simulink model "TCMSSystem"  (R2019b)
settings: configuration reference "ConfigSet_TCMSSystem_Reference" (kept outside this file)
model workspace (MAT data in the model file):
  Prm_TCMSSystem : Simulink.Parameter (value not decoded)
  SampleTime = 0.05
symbols that are objects in the model workspace (value not decoded): Prm_TCMSSystem
undefined symbols (not defined in the file): ADDIntervention, AK1Status, AK2Status, AKContactorStatus, AllDoorsClosed, AllLeftDoorsClosed, AllRightDoorsClosed, APS1Fault, APS1Isolated, APS1OutputVoltage, APS1Status, APS2Fault, APS2Isolated, APS2OutputVoltage, APS2Status, APSKAKContactor, ASCOEnd1, ASCOEnd2, ATBMode, ATCBypassMode, ATCStatusNotOK, ATOMode, ATPLowSpeedCutoutStatus, ATPMode, AuxCompressor, BatteryCurrent, BatteryIsolationContactor, BatteryTemperature, BatteryVoltage, BCG1Fault, BCG1Isolated, BCG1IsolationFailed, BCG1OutputCurrent, BCG1Status, BCG2Fault, BCG2Isolated, BCG2OutputCurrent, BCG2Status, BCGOutputVoltage, BECU1AxleLockedWheelSet1, BECU2AxleLockedWheelSet2, BECUFaulty, BECUMajorFault, BECUMinorFault, BECUStatus, BIC1Inside, BIC1Outside, BIC2Inside, BIC2Outside, Bogie, Bogie1WSPStatus, Bogie2WSPStatus, BogieFaulty, BogieIsolationStatus, BogieSupportedMass, BrakeCylinderPressureGauge, BrakeLoopCBTripped, BrakeLoopOpenTL, BrakeTrainLineStatus, BrakingDemand ... (+215)
libraries: TimersLib x257, simulink x137, LatchesLib x42, VectorOperationsLib x15, TestBenchLib x12, MathOperationsLib x2, FiltersLib x1
(part 3 of 16)

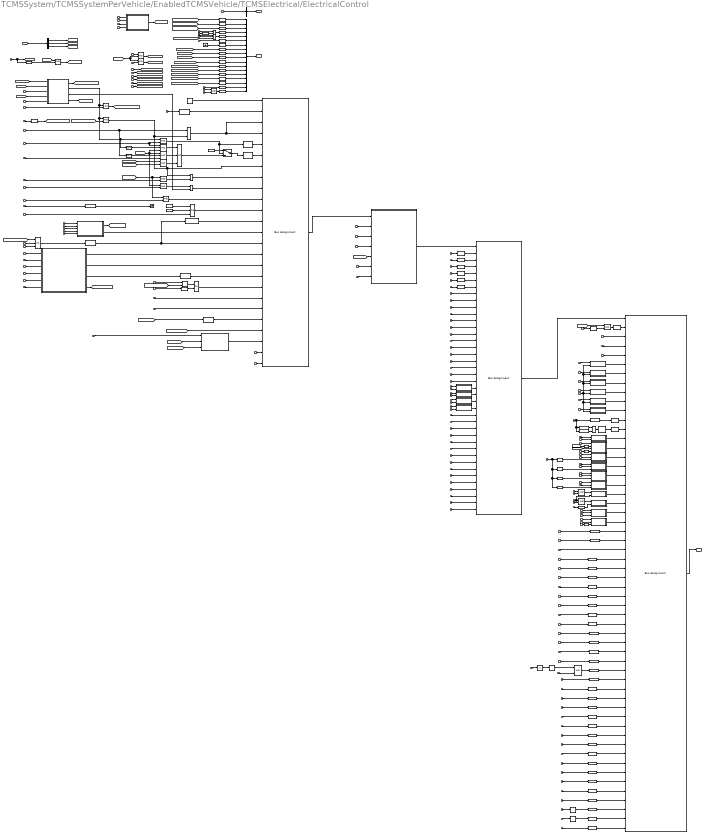
== system TCMSSystem/TCMSSystemPerVehicle/EnabledTCMSVehicle/TCMSElectrical/ElectricalControl ==
  note: Headlight High/Low:
      | Emergency Door Opened
      | Forward direction in UTO Mode
  note: Door Operations
  note: VDUInputs
  note: Fault Message Triggers
  note: Taillight White:
      | In the direction of travel
      | With Mode Selector not in OFF or Standby
  note: Taillight Red:
      | In the opposite direction of travel
      | Emergency door opened at other end
      | In Standstill at both end
  note: Floodlight:
      | Forward direction in UTO Mode
  note: Flashlight:
      | Forward direction in UTO Mode
      | While in RM mode, on the other end
  note: UTO/RM:
      | While in RM mode, on the other end
  note: Call on Light:
      | On the other end
  In Bus Element5 : Inport  PortName=WireStates  Element=TractionBrakingTrainWire.Overspeed
  In Bus Element129 : Inport  PortName=WireStates  Element=ElectricalTrainWire
  In Bus Element12 : Inport  PortName=WireStates  Element=ElectricalTrainWire.TW_EnergizeTLWRFb
  In Bus Element13 : Inport  PortName=WireStates  Element=ElectricalTrainWire.TW_RMF_RMRFb
  In Bus Element6 : Inport  PortName=WireStates  Element=ElectricalTrainWire.TW_PantoDownCmdTrip
  In Bus Element9 : Inport  PortName=WireStates  Element=ElectricalTrainWire.TW_TPOR
  In Bus Element18 : Inport  PortName=WireStates  Element=ElectricalTrainWire.TW_ATPFb
  In Bus Element25 : Inport  PortName=WireStates  Element=ElectricalTrainWire.TW_HLSwitchStatus
  In Bus Element28 : Inport  PortName=WireStates  Element=ElectricalTrainWire.TW_EmerDoorOpened
  In Bus Element26 : Inport  PortName=WireStates  Element=ElectricalTrainWire.TW_CallOnLightStatus
  In Bus Element31 : Inport  PortName=WireStates  Element=ElectricalTrainWire.TW_ZeroSpeed
  In Bus Element32 : Inport  PortName=WireStates  Element=ElectricalTrainWire.TW_UTOModeActive
  In Bus Element34 : Inport  PortName=WireStates  Element=ElectricalTrainWire.TW_DriverModeSelection
  In Bus Element128 : Inport  PortName=WireStates  Element=ElectricalTrainWire.TW_POFFPB
  In Bus Element127 : Inport  PortName=WireStates  Element=ElectricalTrainWire.TW_POFFPB
  In Bus Element130 : Inport  PortName=WireStates  Element=ElectricalTrainWire.TW_ReverseDirection
  In Bus Element132 : Inport  PortName=WireStates  Element=ElectricalTrainWire.TW_KeySwitchStatus
  In Bus Element126 : Inport  PortName=WireStates  Element=ElectricalTrainWire.TW_ShutdownFailure
  In Bus Element153 : Inport  PortName=WireStates  Element=PneumaticTrainSum.NoOfBogieIsolated
  In Bus Element125 : Inport  Port=2  PortName=CBTC
  In Bus Element33 : Inport  Port=2  PortName=CBTC  Element=DriverModeSelection
  In Bus Element45 : Inport  Port=2  PortName=CBTC  Element=ATCWakeup
  In Bus Element124 : Inport  Port=3  PortName=ElectricalSignals
  In Bus Element3 : Inport  Port=3  PortName=ElectricalSignals  Element=CabActive
  In Bus Element114 : Inport  Port=3  PortName=ElectricalSignals  Element=CabActive
  In Bus Element2 : Inport  Port=3  PortName=ElectricalSignals  Element=ZeroSpeed
  In Bus Element7 : Inport  Port=3  PortName=ElectricalSignals  Element=PowerONPBPressed
  In Bus Element8 : Inport  Port=3  PortName=ElectricalSignals  Element=PowerOFFPBPressed
  In Bus Element19 : Inport  Port=3  PortName=ElectricalSignals  Element=ForwardDirection
  In Bus Element22 : Inport  Port=3  PortName=ElectricalSignals  Element=ReverseDirection
  In Bus Element23 : Inport  Port=3  PortName=ElectricalSignals  Element=HLSwitchStatus
  In Bus Element29 : Inport  Port=3  PortName=ElectricalSignals  Element=FlasherLightStatus
  In Bus Element30 : Inport  Port=3  PortName=ElectricalSignals  Element=CallOnLightStatus
  In Bus Element16 : Inport  Port=3  PortName=ElectricalSignals  Element=PADRStatus
  In Bus Element87 : Inport  Port=3  PortName=ElectricalSignals  Element=PADRStatus
  In Bus Element17 : Inport  Port=3  PortName=ElectricalSignals  Element=ParkBrakeApplication
  In Bus Element48 : Inport  Port=3  PortName=ElectricalSignals  Element=BatteryVoltage
  In Bus Element49 : Inport  Port=3  PortName=ElectricalSignals  Element=BUVDR_Active
  In Bus Element50 : Inport  Port=3  PortName=ElectricalSignals  Element=CMCActivationFault
  In Bus Element51 : Inport  Port=3  PortName=ElectricalSignals  Element=CMCDeactivationFault
  In Bus Element52 : Inport  Port=3  PortName=ElectricalSignals  Element=VCBTripCommand
  In Bus Element{62,67..68,86} (4 alike) : Inport  Port=3  PortName=ElectricalSignals  Element=TPOR_ON
  In Bus Element{72,88..89,94} (4 alike) : Inport  Port=3  PortName=ElectricalSignals  Element=UW_VCB
  In Bus Element90 : Inport  Port=3  PortName=ElectricalSignals  Element=PantoDownPBCmd
  In Bus Element69 : Inport  Port=3  PortName=ElectricalSignals  Element=PantoDownPBCmd
  In Bus Element70 : Inport  Port=3  PortName=ElectricalSignals  Element=ADDCOSStatus
  In Bus Element91 : Inport  Port=3  PortName=ElectricalSignals  Element=ORDCOSStatus
  In Bus Element92 : Inport  Port=3  PortName=ElectricalSignals  Element=MRIsolation
  In Bus Element93 : Inport  Port=3  PortName=ElectricalSignals  Element=MCBPAGroupStatus
  In Bus Element97 : Inport  Port=3  PortName=ElectricalSignals  Element=MCB110VDCGroup
  In Bus Element98 : Inport  Port=3  PortName=ElectricalSignals  Element=MCBLightGroup
  In Bus Element99 : Inport  Port=3  PortName=ElectricalSignals  Element=MCBLightSaloonGroup
  In Bus Element100 : Inport  Port=3  PortName=ElectricalSignals  Element=MCBDoorGroup
  In Bus Element101 : Inport  Port=3  PortName=ElectricalSignals  Element=MCBBrakeGroup
  In Bus Element102 : Inport  Port=3  PortName=ElectricalSignals  Element=MCBAPSGroup
  In Bus Element103 : Inport  Port=3  PortName=ElectricalSignals  Element=MCBTCMSGroup
  In Bus Element104 : Inport  Port=3  PortName=ElectricalSignals  Element=MCBSignallingGroup
  In Bus Element105 : Inport  Port=3  PortName=ElectricalSignals  Element=CECBTripped
  In Bus Element106 : Inport  Port=3  PortName=ElectricalSignals  Element=UCCBTripped
  In Bus Element107 : Inport  Port=3  PortName=ElectricalSignals  Element=PANCBTripped
  In Bus Element108 : Inport  Port=3  PortName=ElectricalSignals  Element=ELCB1Tripped
  In Bus Element109 : Inport  Port=3  PortName=ElectricalSignals  Element=ELCB2Tripped
  In Bus Element110 : Inport  Port=3  PortName=ElectricalSignals  Element=ILCB1Tripped
  In Bus Element111 : Inport  Port=3  PortName=ElectricalSignals  Element=ILCB2Tripped
  In Bus Element112 : Inport  Port=3  PortName=ElectricalSignals  Element=APSCBTripped
  In Bus Element113 : Inport  Port=3  PortName=ElectricalSignals  Element=ReverseMotionInForwardCommandMessage
  In Bus Element115 : Inport  Port=3  PortName=ElectricalSignals  Element=MCDRFaulty
  In Bus Element118 : Inport  Port=3  PortName=ElectricalSignals  Element=FwdRevTrainLineMismatchMessage
  In Bus Element119 : Inport  Port=3  PortName=ElectricalSignals  Element=LowMRPressureFaultMessage
  In Bus Element120 : Inport  Port=3  PortName=ElectricalSignals  Element=ObstacleDetected
  In Bus Element121 : Inport  Port=3  PortName=ElectricalSignals  Element=ODDFailure
  In Bus Element10 : Inport  Port=3  PortName=ElectricalSignals  Element=TSDR_ON
  In Bus Element63 : Inport  Port=3  PortName=ElectricalSignals  Element=VCBState
  In Bus Element150 : Inport  Port=3  PortName=ElectricalSignals  Element=VCBState
  In Bus Element131 : Inport  Port=3  PortName=ElectricalSignals  Element=Key_Switch_Status
  In Bus Element151 : Inport  Port=3  PortName=ElectricalSignals  Element=DeadmanBypassStatus
  In Bus Element152 : Inport  Port=3  PortName=ElectricalSignals  Element=BLCOSwitchStatus
  In Bus Element154 : Inport  Port=3  PortName=ElectricalSignals  Element=NoOfEPICCutout
  In Bus Element155 : Inport  Port=3  PortName=ElectricalSignals  Element=WFLIsolated
  In Bus Element171 : Inport  Port=3  PortName=ElectricalSignals  Element=RemoteMagnetValve1
  In Bus Element172 : Inport  Port=3  PortName=ElectricalSignals  Element=RemoteMagnetValve2
  TCMSSystemVehicleConfig : Inport  Port=4
  In Bus Element15 : Inport  Port=5  PortName=Environment
  In Bus Element123 : Inport  Port=5  PortName=Environment  Element=VehiclesPassedNS
  In Bus Element122 : Inport  Port=5  PortName=Environment  Element=NeutralSection
  In Bus Element1 : Inport  Port=6  PortName=DoorSystem  Element=EmergencyDoor.EmergencyDoorOpen
  In Bus Element14 : Inport  Port=6  PortName=DoorSystem  Element=Doors
  In Bus Element20 : Inport  Port=6  PortName=DoorSystem  Element=AllLeftDoorClosed
  In Bus Element21 : Inport  Port=6  PortName=DoorSystem  Element=AllRightDoorClosed
  In Bus Element83 : Inport  Port=7  PortName=DisplayControl
  In Bus Element4 : Inport  Port=7  PortName=DisplayControl  Element=LVCommandPOPB
  In Bus Element11 : Inport  Port=7  PortName=DisplayControl  Element=ParkBrakeReleaseVDUReq
  In Bus Element38 : Inport  Port=7  PortName=DisplayControl  Element=LVIsolateBCG1
  In Bus Element39 : Inport  Port=7  PortName=DisplayControl  Element=LVIsolateBCG2
  In Bus Element : Inport  Port=7  PortName=DisplayControl  Element=ParkBrakeApplyVDUReq
  In Bus Element24 : Inport  Port=7  PortName=DisplayControl  Element=ParkBrakeBypassVDUReq
  In Bus Element27 : Inport  Port=7  PortName=DisplayControl  Element=Bogie1IsolateVDUReq
  In Bus Element35 : Inport  Port=7  PortName=DisplayControl  Element=Bogie2IsolateVDUReq
  In Bus Element37 : Inport  Port=7  PortName=DisplayControl  Element=HornHigh
  In Bus Element40 : Inport  Port=7  PortName=DisplayControl  Element=HornLow
  In Bus Element41 : Inport  Port=7  PortName=DisplayControl  Element=HornIsolate
  In Bus Element77 : Inport  Port=7  PortName=DisplayControl  Element=TCMSIsolatePanto
  In Bus Element78 : Inport  Port=7  PortName=DisplayControl  Element=TCMSIsolateVCB
  In Bus Element79 : Inport  Port=7  PortName=DisplayControl  Element=TCMSIsolateAPS1
  In Bus Element80 : Inport  Port=7  PortName=DisplayControl  Element=TCMSIsolateAPS2
  In Bus Element81 : Inport  Port=7  PortName=DisplayControl  Element=TCMSPantoRiseReq
  In Bus Element82 : Inport  Port=7  PortName=DisplayControl  Element=TCMSPantoLowerReq
  In Bus Element134 : Inport  Port=7  PortName=DisplayControl  Element=TCMSHVAC1ResetReq
  In Bus Element135 : Inport  Port=7  PortName=DisplayControl  Element=TCMSHVAC2ResetReq
  In Bus Element136 : Inport  Port=7  PortName=DisplayControl  Element=TCMSHVAC1IsolateReq
  In Bus Element137 : Inport  Port=7  PortName=DisplayControl  Element=TCMSHVAC2IsolateReq
  In Bus Element138 : Inport  Port=7  PortName=DisplayControl  Element=TCMSHVACSmokeResetReq
  In Bus Element139 : Inport  Port=7  PortName=DisplayControl  Element=TCMSFireAlarmResetReq
  In Bus Element140 : Inport  Port=7  PortName=DisplayControl  Element=TCMSFDUResetReq
  In Bus Element141 : Inport  Port=7  PortName=DisplayControl  Element=TCMSAPSICBOpen
  In Bus Element142 : Inport  Port=7  PortName=DisplayControl  Element=TCMSAPSICBClose
  In Bus Element143 : Inport  Port=7  PortName=DisplayControl  Element=TCMSHVAC1Close
  In Bus Element144 : Inport  Port=7  PortName=DisplayControl  Element=TCMSHVAC1Open
  In Bus Element145 : Inport  Port=7  PortName=DisplayControl  Element=TCMSHVAC2Open
  In Bus Element146 : Inport  Port=7  PortName=DisplayControl  Element=TCMSHVAC2Close
  In Bus Element147 : Inport  Port=7  PortName=DisplayControl  Element=TCMSFDSCBClose
  In Bus Element148 : Inport  Port=7  PortName=DisplayControl  Element=TCMSFDSCBOpen
  In Bus Element156 : Inport  Port=7  PortName=DisplayControl  Element=TCMSWFLIsolationReq
  In Bus Element157 : Inport  Port=7  PortName=DisplayControl  Element=TCMSPABORBypassReq
  In Bus Element158 : Inport  Port=7  PortName=DisplayControl  Element=HVAC1FireDetectorDisableVDUReq
  In Bus Element159 : Inport  Port=7  PortName=DisplayControl  Element=EDBHeatAlarmDisableVDUReq
  In Bus Element160 : Inport  Port=7  PortName=DisplayControl  Element=CABSmokeDetectorDisableVDUReq
  In Bus Element161 : Inport  Port=7  PortName=DisplayControl  Element=SHDEndCubicleRearRight1DisableVDUReq
  In Bus Element162 : Inport  Port=7  PortName=DisplayControl  Element=SHDEndCubicleRearRight2DisableVDUReq
  In Bus Element163 : Inport  Port=7  PortName=DisplayControl  Element=SHDEndCubicleRearLeft1DisableVDUReq
  In Bus Element164 : Inport  Port=7  PortName=DisplayControl  Element=SHDEndCubicleRearLeft2DisableVDUReq
  In Bus Element165 : Inport  Port=7  PortName=DisplayControl  Element=LHDDriverDeskDisableVDUReq
  In Bus Element166 : Inport  Port=7  PortName=DisplayControl  Element=LHDCIDisableVDUReq
  In Bus Element167 : Inport  Port=7  PortName=DisplayControl  Element=LHDLTJBDisableVDUReq
  In Bus Element168 : Inport  Port=7  PortName=DisplayControl  Element=SaloonR1FireDetectorDisableVDUReq
  In Bus Element169 : Inport  Port=7  PortName=DisplayControl  Element=SaloonR2FireDetectorDisableVDUReq
  In Bus Element170 : Inport  Port=7  PortName=DisplayControl  Element=AuxiliaryDeskFireDetectorDisableVDUReq
  In Bus Element36 : Inport  Port=8  PortName=InputControlStates  Element=ControlKey
  In Bus Element42 : Inport  Port=8  PortName=InputControlStates  Element=ControlKey
  In Bus Element43 : Inport  Port=8  PortName=InputControlStates  Element=ModeSelector
  In Bus Element44 : Inport  Port=8  PortName=InputControlStates  Element=TractionBrakeController
  In Bus Element116 : Inport  Port=8  PortName=InputControlStates  Element=DeadManBypass
  In Bus Element46 : Inport  Port=9  PortName=TCMSFaults  Element=NeutralZoneVCBBackupFunctionActivated
  In Bus Element47 : Inport  Port=9  PortName=TCMSFaults  Element=CCUCommunicationError
  In Bus Element53 : Inport  Port=10  PortName=VehicleFaults  Element=OHLHighVoltageLevel3
  In Bus Element54 : Inport  Port=10  PortName=VehicleFaults  Element=OHLLowVoltageLevel2
  In Bus Element55 : Inport  Port=10  PortName=VehicleFaults  Element=VCBOpenedByCI
  In Bus Element56 : Inport  Port=10  PortName=VehicleFaults  Element=VCBOpenedByACOvercurrent
  In Bus Element57 : Inport  Port=10  PortName=VehicleFaults  Element=VCBOpenedByMTrProtection
  In Bus Element58 : Inport  Port=10  PortName=VehicleFaults  Element=VCBOpenedByAPS
  In Bus Element59 : Inport  Port=10  PortName=VehicleFaults  Element=BICContactorActivationFault
  In Bus Element149 : Inport  Port=10  PortName=VehicleFaults  Element=ShutdownFailureVCBOpening
  In Bus Element65 : Inport  Port=10  PortName=VehicleFaults  Element=ShutdownFailureVCBOpening
  In Bus Element60 : Inport  Port=10  PortName=VehicleFaults  Element=PantographLoweringFailure
  In Bus Element64 : Inport  Port=10  PortName=VehicleFaults  Element=PantographRisingMissing
  In Bus Element66 : Inport  Port=10  PortName=VehicleFaults  Element=PantographLoweringMissing
  In Bus Element71 : Inport  Port=10  PortName=VehicleFaults  Element=PantographRisingInhibited
  In Bus Element73 : Inport  Port=10  PortName=VehicleFaults  Element=AKOpenFailure
  In Bus Element74 : Inport  Port=10  PortName=VehicleFaults  Element=KOpenFailure
  In Bus Element84 : Inport  Port=10  PortName=VehicleFaults  Element=VCBMissingClosing
  In Bus Element85 : Inport  Port=10  PortName=VehicleFaults  Element=VCBMissingOpening
  In Bus Element61 : Inport  Port=11  PortName=TractionOut  Element=FilterVoltage
  In Bus Element75 : Inport  Port=11  PortName=TractionOut  Element=TCU_KStatus
  In Bus Element76 : Inport  Port=11  PortName=TractionOut  Element=TCU_AKStatus
  In Bus Element96 : Inport  Port=12  PortName=PantographSignals
  In Bus Element95 : Inport  Port=12  PortName=PantographSignals  Element=PantographPosition
  In Bus Element117 : Inport  Port=13  PortName=ElectricalTrainSum  Element=ControlKey
  In Bus Element133 : Inport  Port=14  PortName=PneumaticsSignals
  AND{,1,3..4,9..19} (15 alike) : Logic  AllPortsSameDT=off  OutDataTypeStr=boolean
  AND2 : Logic  Inputs=3  AllPortsSameDT=off  OutDataTypeStr=boolean
  AND5 : Logic  Inputs=3  AllPortsSameDT=off  OutDataTypeStr=boolean
  AND6 : Logic  Operator=OR  AllPortsSameDT=off  OutDataTypeStr=boolean
  AND7 : Logic  Operator=OR  AllPortsSameDT=off  OutDataTypeStr=boolean
  AND8 : Logic  Operator=OR  Inputs=3  AllPortsSameDT=off  OutDataTypeStr=boolean
  Automatic Start Mode : Subsystem
  Bus Assignment : BusAssignment  AssignedSignals=Overspeed,EnergizeHLHBR,EnergizeHLLBR,EnergizeTLWR,EnergizeTLRR,EnergizeFLDR,EnergizeFLR,EnergizeRM,EnergizeCOLR,PantoDownCmdTrip,TCMS_TPOR,TCMS_TSDR,PantoMVSet,TCMS_VCBClose,TCMS_VCBOpen,NeutralZoneBackupModeActive,TCMS_PBR,VehiclesPassedNS,NeutralSection,TW_TSDDR,TrainInNeutralSection,TCMSCompressorCmd,RemoteMagnetValve1,RemoteMagnetValve2
  Bus Assignment1 : BusAssignment  AssignedSignals=BatteryLowFault,BUVDR_Active,CMCActivationFault,CMCDeactivationFault,OHLHighVoltageLevel3,OHLLowVoltageLevel2,VCBOpenedByCI,VCBOpenedByACOvercurrent,VCBOpenedByMTrProtection,VCBOpenedByAPS,DCLinkOverVoltageLevel1,DCLinkLowVoltageLevel1,BICContactorActivationFault,ShutdownFailureVCBNotOpening,PantographRisingMissing,PantographLoweringMissing,PantographRisingInhibited,PantographLoweringFailure,AKOpenFailure,KOpenFailure,VCBMissingClosing,VCBMissingOpening,FwdRevTrainLineMismatchMessage,LowMRPressureFaultMessage,DeadmanBypass,ADDCOSStatus,ORDCOSStatus,AirSupplyIC,MCBPAGroupStatus,MCB110VDCGroup,MCBLightGroup,MCBLightSaloonGroup,MCBDoorGroup,MCBBrakeGroup,MCBAPSGroup,MCBTCMSGroup,MCBSignallingGroup,DoubleCabKeyInsertion,CabEnableNotEnergized,CouplingCircuitNotEnergized,PantoCircuitNotEnergized,ExternalLightCB1Tripped,ExternalLightCB2Tripped,InternalLightCB1Tripped,InternalLightCB2Tripped,APSCBTripped,ReverseMotionInForwardCommandMessage,MCDRFaulty,ObstacleDetected,ODDFailure,DeadmanBypassStatus,BLCOSwitchStatus,TooManyBogiesIsolated,TooManyEPICCutout,WFLIsolated
  Bus Assignment2 : BusAssignment  AssignedSignals=TCMSIsolateBCG1,TCMSIsolateBCG2,ParkBrakeApplyVDUReq,ParkBrakeBypassVDUReq,Bogie1IsolateVDUReq,Bogie2IsolateVDUReq,HornHighVDUReq,HornLowVDUReq,HornIsolateReinstateVDUReq,TCMSIsolatePanto,TCMSIsolateVCB,TCMSIsolateAPS1,TCMSIsolateAPS2,TCMSFireAlarmReset,TCMSFDUReset,TCMSHVACSmokeReset,TCMSIsolateHVAC1,TCMSIsolateHVAC2,TCMSResetHVAC1,TCMSResetHVAC2,TCMSAPSCBTripCmd,TCMSFDSCBTripCmd,TCMSHVAC1CBTripCmd,TCMSHVAC2CBTripCmd,TCMSWFLIsolation,TCMSPABORBypass,HVAC1FireDetectorDisableVDUReq,EDBHeatAlarmDisableVDUReq,CABSmokeDetectorDisableVDUReq,SHDEndCubicleRearRight1DisableVDUReq,SHDEndCubicleRearRight2DisableVDUReq,SHDEndCubicleRearLeft1DisableVDUReq,SHDEndCubicleRearLeft2DisableVDUReq,LHDDriverDeskDisableVDUReq,LHDCIDisableVDUReq,LHDLTJBDisableVDUReq,SaloonR1FireDetectorDisableVDUReq,SaloonR2FireDetectorDisableVDUReq,AuxiliaryDeskFireDetectorDisableVDUReq
  Bus Creator : BusCreator  Inputs=18  OutDataTypeStr=Bus: BD_TCMSSystem_Wires_ElectricalTrainWire  NonVirtualBus=on
  Bus Creator1 : BusCreator  Inputs=1  OutDataTypeStr=Bus: BD_TCMSSystem_Wires_ElectricalTrainSum  NonVirtualBus=on
  Bus Selector1 : BusSelector  OutputSignals=HasCab,IsMCar,HasVCB
  Compare To Constant : simulink/Logic and Bit Operations/Compare To Constant  relop=<=  const=95  OutDataTypeStr=boolean
  Compare To Constant1 : simulink/Logic and Bit Operations/Compare To Constant  relop=>=  const=2000  OutDataTypeStr=boolean
  Compare To Constant10 : simulink/Logic and Bit Operations/Compare To Constant  relop=>=  const=3.0  OutDataTypeStr=boolean
  Compare To Constant2 : simulink/Logic and Bit Operations/Compare To Constant  relop=<  const=1600  OutDataTypeStr=boolean
  Compare To Constant3 : simulink/Logic and Bit Operations/Compare To Constant  relop=>  const=1000  OutDataTypeStr=boolean
  Compare To Constant4 : simulink/Logic and Bit Operations/Compare To Constant  relop===  const=1  OutDataTypeStr=boolean
  Compare To Constant5 : simulink/Logic and Bit Operations/Compare To Constant  relop===  const=1  OutDataTypeStr=boolean
  Compare To Constant6 : simulink/Logic and Bit Operations/Compare To Constant  relop===  const=0  OutDataTypeStr=boolean
  Compare To Constant7 : simulink/Logic and Bit Operations/Compare To Constant  relop===  const=0  OutDataTypeStr=boolean
  Compare To Constant8 : simulink/Logic and Bit Operations/Compare To Constant  relop=>=  const=2  OutDataTypeStr=boolean
  Compare To Constant9 : simulink/Logic and Bit Operations/Compare To Constant  relop=>=  const=6.0  OutDataTypeStr=boolean
  Compressor_Start_Stop : Subsystem
  Constant : Constant  Value=0
  Constant1 : Constant  Value=0
  Constant2 : Constant  Value=0
  Constant7 : Constant  Value=0  OutDataTypeStr=Bus: BD_TCMSSystem_Out_Vehicle_Control_ElectricalSystem
  Data Type Conversion{,1..64,67} (66 alike) : DataTypeConversion
  Detect Increase : simulink/Logic and Bit Operations/Detect Increase  vinit=0.0  OutDataTypeStr=boolean
  Doors : Subsystem
  Ground1 : Ground
  Logical Operator : Logic  Operator=OR  Inputs=3  AllPortsSameDT=off  OutDataTypeStr=boolean
  Logical Operator1 : Logic  AllPortsSameDT=off  OutDataTypeStr=boolean
  Logical Operator2 : Logic  Operator=NOT  AllPortsSameDT=off  OutDataTypeStr=boolean
  Logical Operator9 : Logic  Operator=NOT  AllPortsSameDT=off  OutDataTypeStr=boolean
  NOT{,1..4} (5 alike) : Logic  Operator=NOT  AllPortsSameDT=off  OutDataTypeStr=boolean
  OR{1..2,4,9} (4 alike) : Logic  Operator=OR  AllPortsSameDT=off  OutDataTypeStr=boolean
  OR3 : Logic  Operator=OR  Inputs=3  AllPortsSameDT=off  OutDataTypeStr=boolean
  OR7 : Logic  Operator=OR  Inputs=3  AllPortsSameDT=off  OutDataTypeStr=boolean
  Subsystem : Subsystem
  Subsystem1 : Subsystem
  Subsystem10 : Subsystem
  Subsystem11 : Subsystem
  Subsystem12 : Subsystem
  Subsystem13 : Subsystem
  Subsystem14 : Subsystem
  Subsystem15 : Subsystem
  Subsystem16 : Subsystem
  Subsystem17 : Subsystem
  Subsystem18 : Subsystem
  Subsystem19 : Subsystem
  Subsystem2 : Subsystem
  Subsystem20 : Subsystem
  Subsystem21 : Subsystem
  Subsystem22 : Subsystem
  Subsystem3 : Subsystem
  Subsystem4 : Subsystem
  Subsystem5 : Subsystem
  Subsystem6 : Subsystem
  Subsystem7 : Subsystem
  Subsystem8 : Subsystem
  Subsystem9 : Subsystem
  Sum of Elements : Sum  Inputs=+
  Switch : Switch  Criteria=u2 > Threshold
  Terminator2 : Terminator
  TimerOffDelay NoInit : TimersLib/TimerOffDelay NoInit  UpperSaturationLimit=1  SampleTime=-1
      settings: SourceProductName=Sydac Utilities
  TimerOnDelay NoInit : TimersLib/TimerOnDelay NoInit  UpperSaturationLimit=4  OutputTime=off  SampleTime=-1
      settings: SourceProductName=Sydac Utilities
  TimerOnDelay NoInit1 : TimersLib/TimerOnDelay NoInit  UpperSaturationLimit=0.05  OutputTime=off  SampleTime=-1
      settings: SourceProductName=Sydac Utilities
  TimerOnDelay NoInit2 : TimersLib/TimerOnDelay NoInit  UpperSaturationLimit=0.05  OutputTime=off  SampleTime=-1
      settings: SourceProductName=Sydac Utilities
  ElectricalTWSources : Outport
  ElectricalTWSumSources : Outport  Port=2
  Control : Outport  Port=3
  wires:
  In Bus Element5/1 -> Data Type Conversion4/1
  Data Type Conversion4/1 -> Bus Assignment/2  "Overspeed"
  Constant7/1 -> Bus Assignment/1  "Control"
  In Bus Element3/1 -> [ActiveCab], NOT/1
  Data Type Conversion/1 -> Bus Creator/1  "TW_EnergizeTLWRFb"
  Bus Creator/1 -> ElectricalTWSources/1
  [HasCab] -> AND5/3, AND3/1, AND2/1
  TCMSSystemVehicleConfig/1 -> Bus Selector1/1
  [TWEnergizeTLWRSource] -> Data Type Conversion/1  "TWEnergizeTLWRSource"
  OR4/1 -> Bus Assignment/8  "EnergizeFLR"
  [TW_RMF_RMR_Source] -> Data Type Conversion1/1  "TW_RMF_RMR_Source"
  In Bus Element29/1 -> [TW_RMF_RMR_Source]
  In Bus Element13/1 -> AND1/2
  Data Type Conversion1/1 -> Bus Creator/2  "TW_RMF_RMRFb"
  NOT/1 -> AND10/2
  [TW_ATP] -> Data Type Conversion2/1  "TW_ATP_Source"
  Data Type Conversion2/1 -> Bus Creator/3  "TW_ATPFb"
  OR7/1 -> Switch/3  "EnergizeTLRR"
  In Bus Element31/1 -> AND2/3  "Standstill"
  In Bus Element16/1 -> OR9/1
  Data Type Conversion5/1 -> Bus Creator/4  "TW_PantoDownCmdTrip"
  In Bus Element6/1 -> Data Type Conversion7/1
  Data Type Conversion7/1 -> Terminator2/1
  In Bus Element7/1 -> OR3/1
  Data Type Conversion6/1 -> Bus Creator/5  "TW_TPOR"
  Data Type Conversion8/1 -> Bus Creator/7  "TW_TSDR"
  In Bus Element9/1 -> AND8/3
  In Bus Element15/1 -> Subsystem/2(Environment)
  AND14/1 -> OR1/2, OR4/1, Bus Assignment/7  "EnergizeHL"
  In Bus Element18/1 -> AND3/2
  Bus Selector1/1 -> [HasCab]  "<HasCab>"
  [HasCab] -> AND10/1
  AND10/1 -> [NonActiveCab]
  AND17/1 -> [ForwardSource]
  AND18/1 -> [ReverseSource]
  [ForwardSource] -> Data Type Conversion11/1
  [ReverseSource] -> Data Type Conversion13/1
  Data Type Conversion11/1 -> Bus Creator/9  "TW_ForwardDirection"
  Data Type Conversion13/1 -> Bus Creator/10  "TW_ReverseDirection"
  In Bus Element23/1 -> [HLSwitchStatusSource]
  [HLSwitchStatusSource] -> Data Type Conversion14/1
  Data Type Conversion14/1 -> Bus Creator/11  "TW_HLSwitchStatus"
  In Bus Element25/1 -> AND7/2
  AND7/1 -> [TWEnergizeTLWRSource]
  In Bus Element12/1 -> AND4/2, AND5/1
  [NonActiveCab] -> AND13/1, AND1/1
  AND1/1 -> OR4/2
  Logical Operator/1 -> Bus Assignment/11
  TimerOffDelay NoInit/1 -> Bus Assignment/12
  Data Type Conversion9/1 -> TimerOffDelay NoInit/1, Bus Assignment/14
  Subsystem/1(VCBC) -> Bus Assignment/15
  Subsystem/2(VCBO) -> Bus Assignment/16
  In Bus Element1/1 -> [EmergencyDoorOpened]
  [EmergencyDoorOpened] -> Data Type Conversion19/1
  Data Type Conversion19/1 -> Bus Creator/12  "TW_EmerDoorOpened"
  AND13/1 -> Bus Assignment/10
  In Bus Element30/1 -> [CallOnLightStatus]
  [CallOnLightStatus] -> Data Type Conversion20/1
  Data Type Conversion20/1 -> Bus Creator/13  "TW_CallOnLightStatus"
  In Bus Element26/1 -> AND13/2
  In Bus Element28/1 -> Logical Operator9/1, OR1/1
  In Bus Element2/1 -> [ZeroSpeed]
  [ZeroSpeed] -> Data Type Conversion22/1
  Data Type Conversion22/1 -> Bus Creator/14  "TW_ZeroSpeed"
  Logical Operator9/1 -> AND2/2
  OR1/1 -> Bus Assignment/3, Bus Assignment/4
  [ATCWakeup] -> Data Type Conversion23/1
  Data Type Conversion23/1 -> Bus Creator/15  "TW_UTOModeActive"
  In Bus Element32/1 -> Data Type Conversion16/1
  In Bus Element33/1 -> [DriverModeSelection]
  [DriverModeSelection] -> Data Type Conversion15/1
  Data Type Conversion15/1 -> Bus Creator/16  "TW_DriverModeSelection"
  AND3/1 -> OR2/1
  OR2/1 -> Bus Assignment/9  "EnergizeRM"
  OR3/1 -> Data Type Conversion6/1
  [TW_UTOModeActiveFb] -> AND14/2
  [TW_UTOModeActiveFb] -> OR3/3
  [TW_UTOModeActiveFb] -> AND9/2
  Data Type Conversion16/1 -> [TW_UTOModeActiveFb]  "TW_DriverModeSelection"
  [NonActiveCab] -> Subsystem1/1(NonActiveCab)
  [HasCab] -> Subsystem1/2(HasCab)
  In Bus Element34/1 -> Subsystem1/3(Mode)
  [ActiveCab] -> Subsystem1/4(ActiveCab)
  Subsystem1/1(ATPMode) -> [TW_ATP]
  Subsystem1/3(RMMode) -> OR2/2
  AND2/1 -> OR7/2
  AND5/1 -> OR7/1
  Logical Operator2/1 -> AND5/2
  In Bus Element11/1 -> Data Type Conversion26/1
  AND6/1 -> Bus Assignment/18
  Data Type Conversion26/1 -> AND6/2
  Subsystem1/4(AutoMode) -> [AutoMode]
  In Bus Element36/1 -> Bus Creator1/1
  Bus Creator1/1 -> ElectricalTWSumSources/1
  In Bus Element42/1 -> Automatic Start Mode/1(Key_Switch)
  In Bus Element43/1 -> Automatic Start Mode/2(MS)
  In Bus Element44/1 -> Automatic Start Mode/3(TBC)
  AND8/1 -> Data Type Conversion9/1
  [TW_UTOModeActiveFb] -> AND8/1
  Automatic Start Mode/1(AutoStart) -> [ATCWakeup]
  In Bus Element45/1 -> Automatic Start Mode/4(WakeUp)
  In Bus Element46/1 -> Subsystem/3(Fault)
  Subsystem/3(BackupModeActive) -> Data Type Conversion30/1
  Data Type Conversion30/1 -> Bus Assignment/17
  AND9/1 -> AND6/1
  In Bus Element17/1 -> AND9/1
  OR9/1 -> Data Type Conversion5/1
  In Bus Element47/1 -> Detect Increase/1
  Detect Increase/1 -> OR9/2
  Bus Assignment1/1 -> Control/1
  In Bus Element49/1 -> Bus Assignment1/3
  In Bus Element51/1 -> Bus Assignment1/5
  Compare To Constant/1 -> AND/2
  In Bus Element48/1 -> Compare To Constant/1
  Data Type Conversion31/1 -> Bus Assignment1/2
  In Bus Element50/1 -> Bus Assignment1/4
  Bus Assignment2/1 -> Bus Assignment1/1
  In Bus Element27/1 -> Data Type Conversion28/1
  In Bus Element39/1 -> Data Type Conversion24/1
  In Bus Element24/1 -> Data Type Conversion27/1
  Data Type Conversion29/1 -> Bus Assignment2/7
  Data Type Conversion28/1 -> Bus Assignment2/6
  In Bus Element35/1 -> Data Type Conversion29/1
  Data Type Conversion21/1 -> Bus Assignment2/2
  Data Type Conversion24/1 -> Bus Assignment2/3
  In Bus Element/1 -> Data Type Conversion25/1
  In Bus Element38/1 -> Data Type Conversion21/1
  Data Type Conversion25/1 -> Bus Assignment2/4
  Data Type Conversion27/1 -> Bus Assignment2/5
  In Bus Element37/1 -> Bus Assignment2/8
  In Bus Element41/1 -> Bus Assignment2/10
  In Bus Element40/1 -> Bus Assignment2/9
  Bus Assignment/1 -> Doors/1(BusIn)  "Control"
  In Bus Element20/1 -> Doors/2(AllLeftDoorsClosed)  "AllLeftDoorsClosed"
  In Bus Element14/1 -> Doors/3(Unused)
  In Bus Element21/1 -> Doors/4(AllRightDoorsClosed)  "AllRightDoorsClosed"
  [AutoMode] -> Doors/5(AutoMode)
  Doors/1(BusOut) -> Bus Assignment2/1
  In Bus Element53/1 -> Subsystem3/1(Fault)
  In Bus Element52/1 -> Subsystem8/2(VCB), Subsystem7/2(VCB), Subsystem4/2(LV), Subsystem3/2(LV), Subsystem5/2(VCB), Subsystem6/2(VCB)
  Subsystem3/1(Trig) -> Bus Assignment1/6
  Subsystem4/1(Trig) -> Bus Assignment1/7
  In Bus Element54/1 -> Subsystem4/1(Fault)
  Subsystem5/1(Trig) -> Bus Assignment1/8
  In Bus Element55/1 -> Subsystem5/1(Fault)
  Subsystem6/1(Trig) -> Bus Assignment1/9
  Subsystem7/1(Trig) -> Bus Assignment1/10
  Subsystem8/1(Trig) -> Bus Assignment1/11
  In Bus Element56/1 -> Subsystem6/1(Fault)
  In Bus Element57/1 -> Subsystem7/1(Fault)
  In Bus Element58/1 -> Subsystem8/1(Fault)
  Compare To Constant1/1 -> Data Type Conversion3/1
  In Bus Element61/1 -> Compare To Constant3/1, Compare To Constant2/1, Compare To Constant1/1
  Logical Operator1/1 -> TimerOnDelay NoInit/1
  Compare To Constant2/1 -> Logical Operator1/1
  Compare To Constant3/1 -> Logical Operator1/2
  TimerOnDelay NoInit/1 -> Data Type Conversion12/1
  Data Type Conversion3/1 -> Bus Assignment1/12
  Data Type Conversion12/1 -> Bus Assignment1/13
  Bus Selector1/2 -> [IsMCar]  "<IsMCar>"
  AND/1 -> Data Type Conversion31/1
  [IsMCar] -> AND/1
  Subsystem9/1(Trig) -> Bus Assignment1/14
  In Bus Element59/1 -> Subsystem9/1(Fault)
  In Bus Element62/1 -> Subsystem9/2(Cond)
  Subsystem1/2(DrivingDirection) -> AND4/1, Logical Operator2/1, AND14/1, AND7/1
  [NonActiveCab] -> AND11/1
  AND11/1 -> OR7/3
  TimerOnDelay NoInit1/1 -> Bus Assignment/6
  AND4/1 -> Switch/2, TimerOnDelay NoInit2/1
  [AutoMode] -> AND11/2
  TimerOnDelay NoInit2/1 -> Bus Assignment/5
  In Bus Element96/1 -> Subsystem/4(PantographSystem)
  In Bus Element127/1 -> Subsystem10/1(Fault)
  [TSDDR] -> NOT4/1
  Subsystem10/1(Trig) -> Bus Assignment1/15
  In Bus Element67/1 -> Subsystem11/2(Cond)
  In Bus Element71/1 -> Subsystem13/1(Fault)
  In Bus Element69/1 -> Subsystem14/2(Cond)
  In Bus Element90/1 -> Subsystem12/2(Cond)
  In Bus Element66/1 -> Subsystem12/1(Fault)
  In Bus Element60/1 -> Subsystem14/1(Fault)
  Subsystem14/1(Trig) -> Bus Assignment1/19
  In Bus Element68/1 -> Subsystem13/2(Cond)
  Subsystem12/1(Trig) -> Bus Assignment1/17
  In Bus Element64/1 -> Subsystem11/1(Fault)
  Subsystem11/1(Trig) -> Bus Assignment1/16
  Subsystem13/1(Trig) -> Bus Assignment1/18
  In Bus Element72/1 -> NOT1/1
  In Bus Element73/1 -> AND12/1
  In Bus Element74/1 -> AND15/2
  NOT1/1 -> Subsystem16/2(Cond)
  AND12/1 -> Subsystem15/1(Fault)
  AND15/1 -> Subsystem16/1(Fault)
  In Bus Element76/1 -> AND12/2
  In Bus Element75/1 -> Subsystem15/2(Cond), AND15/1
  Subsystem15/1(Trig) -> Bus Assignment1/20
  Subsystem16/1(Trig) -> Bus Assignment1/21
  In Bus Element80/1 -> Bus Assignment2/14
  In Bus Element79/1 -> Bus Assignment2/13
  In Bus Element78/1 -> Bus Assignment2/12
  In Bus Element77/1 -> Bus Assignment2/11
  In Bus Element82/1 -> Logical Operator/3
  In Bus Element81/1 -> AND8/2
  In Bus Element83/1 -> Subsystem/5(DisplayControl)
  Constant/1 -> Logical Operator/1
  Constant1/1 -> Logical Operator/2
  Subsystem17/1(Trig) -> Bus Assignment1/22
  Subsystem18/1(Trig) -> Bus Assignment1/23
  In Bus Element85/1 -> Subsystem18/1(Fault)
  In Bus Element84/1 -> Subsystem17/1(Fault)
  In Bus Element86/1 -> Subsystem17/2(Cond)
  In Bus Element87/1 -> Subsystem18/2(Cond)
  In Bus Element88/1 -> Subsystem17/3(Cond1)
  NOT2/1 -> Subsystem18/3(Cond1)
  In Bus Element89/1 -> NOT2/1
  Compare To Constant4/1 -> Subsystem11/3(Cond1)
  Compare To Constant6/1 -> Subsystem12/3(Cond1)
  Compare To Constant5/1 -> Subsystem13/3(Cond1)
  Compare To Constant7/1 -> Subsystem14/3(Cond1)
  In Bus Element94/1 -> NOT3/1
  NOT3/1 -> Subsystem10/4(Reset)
  In Bus Element95/1 -> Compare To Constant7/1, Compare To Constant5/1, Compare To Constant6/1, Compare To Constant4/1
  In Bus Element92/1 -> Data Type Conversion17/1
  Data Type Conversion41/1 -> Bus Assignment1/40
  Sum of Elements/1 -> Compare To Constant8/1
  Data Type Conversion39/1 -> Bus Assignment1/35
  In Bus Element100/1 -> Data Type Conversion34/1
  Data Type Conversion17/1 -> Bus Assignment1/29
  Data Type Conversion33/1 -> Bus Assignment1/33
  In Bus Element93/1 -> Data Type Conversion32/1
  In Bus Element111/1 -> Data Type Conversion47/1
  In Bus Element116/1 -> Bus Assignment1/26
  In Bus Element99/1 -> Data Type Conversion33/1
  Data Type Conversion44/1 -> Bus Assignment1/43
  Data Type Conversion49/1 -> Bus Assignment1/48
  In Bus Element101/1 -> Data Type Conversion39/1
  Data Type Conversion37/1 -> Bus Assignment1/37
  In Bus Element102/1 -> Data Type Conversion40/1
  In Bus Element109/1 -> Data Type Conversion45/1
  Data Type Conversion40/1 -> Bus Assignment1/36
  Data Type Conversion46/1 -> Bus Assignment1/42
  AND16/1 -> Data Type Conversion18/1
  Data Type Conversion45/1 -> Bus Assignment1/44
  Data Type Conversion38/1 -> Bus Assignment1/38
  In Bus Element113/1 -> Data Type Conversion49/1
  Data Type Conversion48/1 -> Bus Assignment1/47
  In Bus Element107/1 -> Data Type Conversion46/1
  In Bus Element106/1 -> Data Type Conversion42/1
  Data Type Conversion18/1 -> Bus Assignment1/39
  In Bus Element103/1 -> Data Type Conversion37/1
  In Bus Element98/1 -> Data Type Conversion36/1
  Data Type Conversion43/1 -> Bus Assignment1/45
  Compare To Constant8/1 -> AND16/1
  In Bus Element105/1 -> Data Type Conversion41/1
  In Bus Element110/1 -> Data Type Conversion43/1
  In Bus Element97/1 -> Data Type Conversion35/1
  In Bus Element104/1 -> Data Type Conversion38/1
  Data Type Conversion35/1 -> Bus Assignment1/31
  In Bus Element108/1 -> Data Type Conversion44/1
  In Bus Element112/1 -> Data Type Conversion48/1
  Data Type Conversion47/1 -> Bus Assignment1/46
  Data Type Conversion42/1 -> Bus Assignment1/41
  Data Type Conversion52/1 -> Bus Assignment1/28
  In Bus Element91/1 -> Data Type Conversion52/1
  Data Type Conversion51/1 -> Bus Assignment1/27
  In Bus Element114/1 -> AND16/2
  Data Type Conversion32/1 -> Bus Assignment1/30
  Data Type Conversion34/1 -> Bus Assignment1/34
  In Bus Element117/1 -> Sum of Elements/1
  Data Type Conversion36/1 -> Bus Assignment1/32
  In Bus Element70/1 -> Data Type Conversion51/1
  In Bus Element118/1 -> Data Type Conversion53/1
  Data Type Conversion53/1 -> Bus Assignment1/24
  In Bus Element119/1 -> Data Type Conversion54/1
  Data Type Conversion54/1 -> Bus Assignment1/25
  In Bus Element115/1 -> Data Type Conversion55/1
  Data Type Conversion55/1 -> Bus Assignment1/49
  In Bus Element120/1 -> Data Type Conversion50/1
  In Bus Element121/1 -> Data Type Conversion56/1
  Data Type Conversion50/1 -> Bus Assignment1/50
  Data Type Conversion56/1 -> Bus Assignment1/51
  In Bus Element123/1 -> Bus Assignment/19
  In Bus Element122/1 -> Bus Assignment/20
  In Bus Element4/1 -> OR3/2
  Data Type Conversion57/1 -> Bus Creator/8  "TW_TSDDR"
  [TSDDR] -> Data Type Conversion59/1
  Data Type Conversion58/1 -> Bus Creator/6  "TW_POFFPB"
  Ground1/1 -> Data Type Conversion8/1
  In Bus Element128/1 -> Subsystem2/1(TW_POFF)
  In Bus Element10/1 -> Subsystem2/2(TSDR_ON)
  Subsystem2/2(TCMS_TSDR) -> Bus Assignment/13
  Subsystem2/1(TSDDR) -> [TSDDR]
  [TSDDR] -> Data Type Conversion57/1
  In Bus Element124/1 -> Doors/6(ElectricalSignals)
  In Bus Element125/1 -> Doors/7(CBTC)
  Subsystem/4(TrainInNeutralSection) -> [TrainInNeutralSection]
  [TrainInNeutralSection] -> Bus Assignment/22
  In Bus Element129/1 -> Subsystem/1(WireStates)
  In Bus Element63/1 -> Subsystem/6(VCBState)
  In Bus Element130/1 -> Subsystem1/5(TW_ReverseDirection)
  In Bus Element19/1 -> AND17/1
  In Bus Element22/1 -> AND18/2
  [ActiveCab] -> AND18/1, AND17/2
  Constant2/1 -> Switch/1
  Switch/1 -> TimerOnDelay NoInit1/1
  Data Type Conversion10/1 -> Bus Creator/17  "TW_KeySwitchStatus"
  In Bus Element131/1 -> Data Type Conversion10/1
  In Bus Element132/1 -> Subsystem2/3(KeySwitchStatus)
  In Bus Element8/1 -> Data Type Conversion58/1
  In Bus Element133/1 -> Compressor_Start_Stop/1(PneumaticsSignals)
  [ActiveCab] -> Compressor_Start_Stop/2(ActiveCab)
  [NonActiveCab] -> Compressor_Start_Stop/3(NonActiveCab)
  Compressor_Start_Stop/1(CompressorCmd) -> Bus Assignment/23
  In Bus Element139/1 -> Bus Assignment2/15
  In Bus Element140/1 -> Bus Assignment2/16
  In Bus Element138/1 -> Bus Assignment2/17
  In Bus Element136/1 -> Bus Assignment2/18
  In Bus Element137/1 -> Bus Assignment2/19
  In Bus Element134/1 -> Bus Assignment2/20
  In Bus Element135/1 -> Bus Assignment2/21
  Subsystem19/1(Trig) -> Bus Assignment2/22
  Subsystem20/1(Trig) -> Bus Assignment2/24
  Subsystem21/1(Trig) -> Bus Assignment2/25
  In Bus Element147/1 -> Subsystem22/2(Close)
  In Bus Element148/1 -> Subsystem22/1(Open)
  In Bus Element146/1 -> Subsystem21/2(Close)
  In Bus Element145/1 -> Subsystem21/1(Open)
  In Bus Element144/1 -> Subsystem20/1(Open)
  In Bus Element143/1 -> Subsystem20/2(Close)
  In Bus Element142/1 -> Subsystem19/2(Close)
  In Bus Element141/1 -> Subsystem19/1(Open)
  Subsystem22/1(Trig) -> Bus Assignment2/23
  In Bus Element149/1 -> Subsystem2/4(ShutdownFailure)
  Data Type Conversion59/1 -> Bus Assignment/21
  NOT4/1 -> Subsystem10/2(Cond)
  Bus Selector1/3 -> [HasVCB]  "<HasVCB>"
  [HasVCB] -> Subsystem10/3(HasVCB)
  AND19/1 -> Data Type Conversion60/1
  Data Type Conversion60/1 -> Bus Creator/18  "TW_ShutdownFailure"
  In Bus Element126/1 -> Subsystem2/5(TW_ShutdownFailure)
  In Bus Element65/1 -> AND19/1
  In Bus Element150/1 -> AND19/2
  In Bus Element151/1 -> Data Type Conversion61/1
  In Bus Element152/1 -> Data Type Conversion62/1
  Data Type Conversion61/1 -> Bus Assignment1/52
  Data Type Conversion62/1 -> Bus Assignment1/53
  In Bus Element153/1 -> Compare To Constant9/1
  Compare To Constant9/1 -> Data Type Conversion63/1
  Data Type Conversion63/1 -> Bus Assignment1/54
  Compare To Constant10/1 -> Data Type Conversion64/1
  Data Type Conversion64/1 -> Bus Assignment1/55
  In Bus Element154/1 -> Compare To Constant10/1
  In Bus Element156/1 -> Bus Assignment2/26
  In Bus Element157/1 -> Bus Assignment2/27
  In Bus Element155/1 -> Data Type Conversion67/1
  Data Type Conversion67/1 -> Bus Assignment1/56
  In Bus Element158/1 -> Bus Assignment2/28
  In Bus Element159/1 -> Bus Assignment2/29
  In Bus Element160/1 -> Bus Assignment2/30
  In Bus Element161/1 -> Bus Assignment2/31
  In Bus Element162/1 -> Bus Assignment2/32
  In Bus Element163/1 -> Bus Assignment2/33
  In Bus Element164/1 -> Bus Assignment2/34
  In Bus Element165/1 -> Bus Assignment2/35
  In Bus Element166/1 -> Bus Assignment2/36
  In Bus Element167/1 -> Bus Assignment2/37
  In Bus Element168/1 -> Bus Assignment2/38
  In Bus Element169/1 -> Bus Assignment2/39
  In Bus Element170/1 -> Bus Assignment2/40
  In Bus Element172/1 -> Bus Assignment/25
  In Bus Element171/1 -> Bus Assignment/24

== system TCMSSystem/TCMSSystemPerVehicle/EnabledTCMSVehicle/TCMSElectrical/ElectricalDisplay ==
  In Bus Element : Inport  PortName=TCMSSystemVehicleConfig
  In Bus Element9 : Inport  PortName=TCMSSystemVehicleConfig
  In Bus Element20 : Inport  PortName=TCMSSystemVehicleConfig
  CommonVehicleConfig : Inport  Port=2
  In Bus Element{1..2,8,10..11,14,18,21,25,39,42..46,71} (16 alike) : Inport  Port=3  PortName=ElectricalSignals
  In Bus Element26 : Inport  Port=4  PortName=InputControlStates
  In Bus Element5 : Inport  Port=4  PortName=InputControlStates
  In Bus Element6 : Inport  Port=5  PortName=CBTC
  In Bus Element16 : Inport  Port=5  PortName=CBTC
  In Bus Element{4,7,17,19} (4 alike) : Inport  Port=6  PortName=VehicleFaults
  In Bus Element3 : Inport  Port=7  PortName=CouplingSystem
  In Bus Element12 : Inport  Port=8  PortName=TractionFB
  In Bus Element13 : Inport  Port=9  PortName=PantographSignals
  In Bus Element15 : Inport  Port=10  PortName=WireStates
  APSScreen : Subsystem
  BatteryScreen : Subsystem
  BrakeLoopInterlock : Subsystem
  BrakeScreen : Subsystem
  Constant7 : Constant  Value=0  OutDataTypeStr=Bus: BD_TCMSSystem_Out_Vehicle_Display_ElectricalSystem
  EBLoopInterlockScreen : Subsystem
  EnableToRunScreen : Subsystem
  FireDetectionScreen : Subsystem
  FireDetectorScreen : Subsystem
  HVACScreen : Subsystem
  LightsScreen : Subsystem
  LowVoltageScreen : Subsystem
  MediumVoltageScreen : Subsystem
  MiscellaneaScreen : Subsystem
  OperatingandHeaderScreen : Subsystem
  PantographInterlockScreen : Subsystem
  VCBInterlockScreen : Subsystem
  WFLScreen : Subsystem
  Display : Outport
  wires:
  In Bus Element71/1 -> WFLScreen/2(ElectricalSignals)
  WFLScreen/1(BusOut) -> FireDetectionScreen/1(BusIn)
  FireDetectionScreen/1(BusOut) -> HVACScreen/1(BusIn)
  In Bus Element45/1 -> HVACScreen/2(ElectricalSignals)
  HVACScreen/1(BusOut) -> LightsScreen/1(BusIn)
  In Bus Element46/1 -> LightsScreen/2(ElectricalSignals)
  LightsScreen/1(BusOut) -> LowVoltageScreen/1(BusIn)
  In Bus Element43/1 -> LowVoltageScreen/2(ElectricalSignals)
  LowVoltageScreen/1(BusOut) -> MediumVoltageScreen/1(BusIn)
  MediumVoltageScreen/1(BusOut) -> PantographInterlockScreen/1(BusIn)
  PantographInterlockScreen/1(BusOut) -> VCBInterlockScreen/1(BusIn)
  VCBInterlockScreen/1(BusOut) -> EBLoopInterlockScreen/1(BusIn)
  FireDetectorScreen/1(BusOut) -> Display/1  "Display"
  In Bus Element44/1 -> EBLoopInterlockScreen/2(ElectricalSignals)
  In Bus Element26/1 -> EBLoopInterlockScreen/3(InputControls)
  In Bus Element25/1 -> VCBInterlockScreen/2(ElectricalSignals)
  In Bus Element42/1 -> MediumVoltageScreen/2(ElectricalSignals)
  In Bus Element39/1 -> BatteryScreen/2(ElectricalSignals)
  BatteryScreen/1(BusOut) -> WFLScreen/1(BusIn)
  APSScreen/1(BusOut) -> BatteryScreen/1(BusIn)
  In Bus Element10/1 -> APSScreen/2(ElectricalSignals)
  BrakeScreen/1(BusOut) -> APSScreen/1(BusIn)
  In Bus Element8/1 -> BrakeScreen/2(ElectricalSignals)
  Constant7/1 -> OperatingandHeaderScreen/1(BusIn)  "Display"
  OperatingandHeaderScreen/1(BusOut) -> BrakeScreen/1(BusIn)
  In Bus Element2/1 -> OperatingandHeaderScreen/3(ElectricalSignals)
  In Bus Element5/1 -> OperatingandHeaderScreen/4(InputControlStates)
  In Bus Element6/1 -> OperatingandHeaderScreen/5(CBTC)
  In Bus Element/1 -> OperatingandHeaderScreen/2(TCMSSystemVehicleConfig)
  In Bus Element1/1 -> FireDetectionScreen/3(ElectricalSignals)
  In Bus Element4/1 -> VCBInterlockScreen/3(VehicleFaults)
  In Bus Element7/1 -> OperatingandHeaderScreen/6(VehicleFaults)
  In Bus Element3/1 -> OperatingandHeaderScreen/7(CouplingSystem)
  CommonVehicleConfig/1 -> OperatingandHeaderScreen/8(CommonVehicleConfig)
  In Bus Element9/1 -> FireDetectionScreen/2(CommonConfig)
  EBLoopInterlockScreen/1(BusOut) -> EnableToRunScreen/1(BusIn)  "Display"
  EnableToRunScreen/1(BusOut) -> BrakeLoopInterlock/1(BusIn)  "Display"
  BrakeLoopInterlock/1(BusOut) -> MiscellaneaScreen/1(BusIn)  "Display"
  In Bus Element11/1 -> MiscellaneaScreen/2(ElectricalSignals)
  In Bus Element12/1 -> MiscellaneaScreen/3(TractionSignals)
  In Bus Element13/1 -> BrakeLoopInterlock/2(PantographSignals)
  In Bus Element16/1 -> EnableToRunScreen/3(CBTC)
  In Bus Element15/1 -> EnableToRunScreen/4(WireStates)
  In Bus Element14/1 -> EnableToRunScreen/2(ElectricalSignals)
  In Bus Element17/1 -> HVACScreen/3(VehicleFaults)
  In Bus Element18/1 -> BrakeLoopInterlock/3(ElectricalTrainWire)
  In Bus Element19/1 -> MiscellaneaScreen/4(VehicleFaults)
  In Bus Element20/1 -> EBLoopInterlockScreen/4(TCMSSystemVehicleConfig)
  MiscellaneaScreen/1(BusOut) -> FireDetectorScreen/1(BusIn)  "Display"
  In Bus Element21/1 -> FireDetectorScreen/2(ElectricalSignals)

== system TCMSSystem/TCMSSystemPerVehicle/EnabledTCMSVehicle/TCMSPantograph/PantographControl ==
  In Bus Element : Inport  PortName=DisplayControl  Element=TCMSIsolatePanto
  Bus Assignment : BusAssignment  AssignedSignals=PantoIsolationCommand
  Constant7 : Constant  Value=0  OutDataTypeStr=Bus: BD_TCMSSystem_Out_Vehicle_Control_PantographSystem
  Data Type Conversion4 : DataTypeConversion  OutDataTypeStr=boolean
  Control : Outport
  wires:
  In Bus Element/1 -> Data Type Conversion4/1
  Constant7/1 -> Bus Assignment/1  "Control"
  Bus Assignment/1 -> Control/1  "Control"
  Data Type Conversion4/1 -> Bus Assignment/2  "PantoIsolationCommand"

== system TCMSSystem/TCMSSystemPerVehicle/EnabledTCMSVehicle/TCMSPantograph/PantographDisplay ==
  TCMSSystemVehicleConfig : Inport
  ElectricalSignals : Inport  Port=2
  PantographSystem : Inport  Port=3
  Bus Assignment : BusAssignment  AssignedSignals=UnitAtLeastOnePantoUp,UnitAllPantoDown,UnitPantoPowerDetected,VehiclePantoUp,VehiclePantoDown,PantographIsolated,VehiclePantoRising,VehiclePantoLowering,PantographPosition,PantographFault,PantoADDFaultMessage,PantoORDFaultMessage,PantoRaiseFailureMessage
  Bus Selector : BusSelector  OutputSignals=UnitAtLeastOnePantoUp,UnitAllPantoDown,UnitPantoPowerDetected
  Bus Selector1 : BusSelector  OutputSignals=VehiclePantoUp,VehiclePantoDown,VehiclePantoIsolated,VehiclePantoRising,VehiclePantoLowering,PantographPosition,PantographFault,PantoADDFaultMessage,PantoORDFaultMessage,PantoRaiseFailureMessage
  CabUnitDisplay : Subsystem
  Constant7 : Constant  Value=0  OutDataTypeStr=Bus: BD_TCMSSystem_Out_Vehicle_Display_PantographSystem
  TCMSVehicleInfo : Subsystem
  Display : Outport
  wires:
  Constant7/1 -> Bus Assignment/1  "Display"
  Bus Assignment/1 -> Display/1  "Display"
  TCMSSystemVehicleConfig/1 -> CabUnitDisplay/1(TCMSConfig)
  ElectricalSignals/1 -> CabUnitDisplay/2(ElectricalSignals)
  CabUnitDisplay/1(CabUnitDisplay) -> Bus Selector/1  "CabUnitDisplay"
  Bus Selector/3 -> Bus Assignment/4  "<UnitPantoPowerDetected>"
  Bus Selector/2 -> Bus Assignment/3  "<UnitAllPantoDown>"
  Bus Selector/1 -> Bus Assignment/2  "<UnitAtLeastOnePantoUp>"
  PantographSystem/1 -> TCMSVehicleInfo/1(PantographSystem)
  TCMSVehicleInfo/1(TCMSVehicleInfo) -> Bus Selector1/1  "TCMSVehicleInfo"
  Bus Selector1/1 -> Bus Assignment/5  "<VehiclePantoUp>"
  Bus Selector1/2 -> Bus Assignment/6  "<VehiclePantoDown>"
  Bus Selector1/3 -> Bus Assignment/7  "<VehiclePantoIsolated>"
  Bus Selector1/4 -> Bus Assignment/8  "<VehiclePantoRising>"
  Bus Selector1/5 -> Bus Assignment/9  "<VehiclePantoLowering>"
  Bus Selector1/7 -> Bus Assignment/11  "<PantographFault>"
  Bus Selector1/6 -> Bus Assignment/10  "<PantographPosition>"
  Bus Selector1/8 -> Bus Assignment/12  "<PantoADDFaultMessage>"
  Bus Selector1/9 -> Bus Assignment/13  "<PantoORDFaultMessage>"
  Bus Selector1/10 -> Bus Assignment/14  "<PantoRaiseFailureMessage>"
